simulink model "Interface_Model"  (R2017b)
settings: Solver=FixedStepDiscrete  StartTime=0.0  StopTime=inf  RelTol=1e-3  EnableMultiTasking=on
InitFcn:
  | modelSettings
undefined symbols (not defined in the file or in its folder): ip
libraries: gm_combinedTxRx_ExternalMode_lib x3
settings Model: SimulationMode=external  Creator=tcollins  LastModifiedBy=tcollins
settings SolverCC: PositivePriorityOrder=on
settings OptimizationCC: BlockReduction=off  ConditionallyExecuteInputs=off  PassReuseOutputArgsAs=Individual arguments  MaxStackSize=64
settings DebuggingCC: AlgebraicLoopMsg=error  SingleTaskRateTransMsg=error  ParameterTunabilityLossMsg=error
settings HardwareCC: ProdBitPerPointer=32  ProdBitPerSizeT=32  ProdBitPerPtrDiffT=32  ProdLargestAtomicInteger=Long  ProdLargestAtomicFloat=Double  ProdWordSize=32  ProdLongLongMode=on  ProdHWDeviceType=ARM Compatible->ARM Cortex  TargetLargestAtomicInteger=Long  TargetLargestAtomicFloat=Double  TargetIntDivRoundTo=Zero  TargetEndianess=LittleEndian  TargetHWDeviceType=ARM Compatible->ARM Cortex
settings SFSimCC: MATLABDynamicMemAlloc=off
settings RTWCC: SystemTargetFile=ert.tlc  HardwareBoard=Xilinx Zynq-7000 Based IIO Radio  TemplateMakefile=ert_default_tmf  Toolchain=Xilinx Software Development Kit (SDK)  IncludeHyperlinkInReport=on
settings CodeAppCC: ForceParamTrailComments=on  IgnoreCustomStorageClasses=off  OperatorAnnotations=on  SimulinkDataObjDesc=on  SFDataObjDesc=on  InsertBlockDesc=on

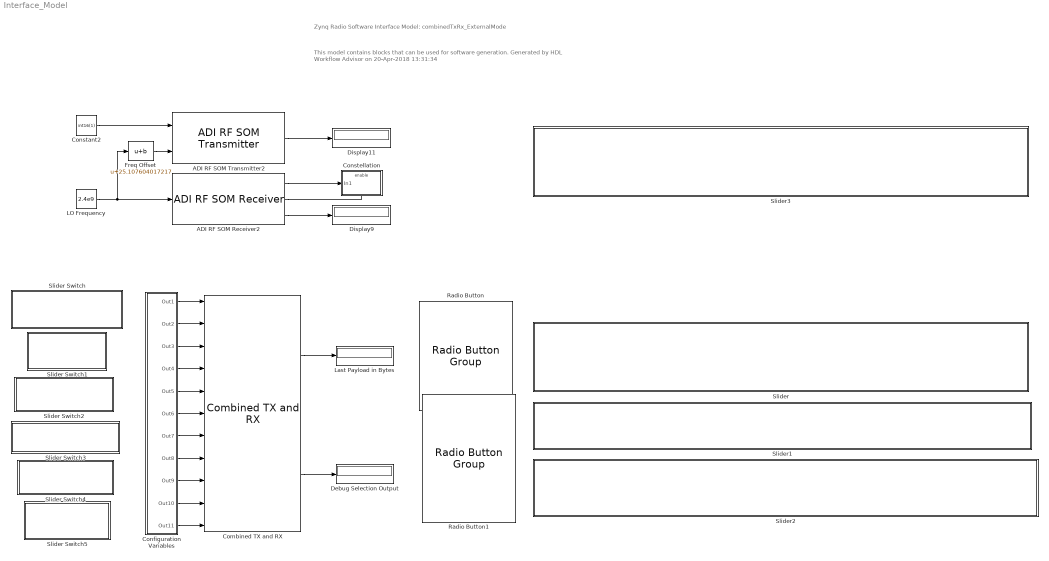
== system Interface_Model ==
  note: Zynq Radio Software Interface Model: combinedTxRx_ExternalMode
  note: This model contains blocks that can be used for software generation.
      |
      | Generated by HDL Workflow Advisor on 20-Apr-2018 13:31:34
  ADI RF SOM Receiver2 : gm_combinedTxRx_ExternalMode_lib/ADI RF SOM Receiver  IPAddress=192.168.3.2  uri=ip:10.0.0.200  CenterFrequencySource=Input Port  CenterFrequency=2.4e9  GainSource=AGC Slow Attack  Gain=10  ChannelMapping=1  BasebandSampleRate=1e6  OutputDataType=int16  SamplesPerFrame=20000  OverflowOutputPort=on  ShowAdvancedProperties=off  Timeout=30  EnableQuadratureTracking=on  EnableRFDCTracking=on  EnableBasebandDCTracking=on  UseCustomFilter=off  filtPathRates=[ 737280000, 11520000, 3840000, 1920000, 960000, 240000 ]  filtCoefficients=round( fir1( 127, 0.75 )*2^15*10^1.2 )  filtCoefficientSize=128  filtDecimInterpFactor=4  filtGain=-12  filtRFBandwidth=18e6  filterConfigStruct=struct()  ENSMPinControlMode=None  BISTLoopbackMode=Disabled
  ADI RF SOM Transmitter2 : gm_combinedTxRx_ExternalMode_lib/ADI RF SOM Transmitter  IPAddress=192.168.3.2  uri=ip:10.0.0.200  CenterFrequencySource=Input Port  CenterFrequency=2.4e9  GainSource=Dialog  Gain=-10  ChannelMapping=1  BasebandSampleRate=1e6  UnderflowOutputPort=on  ShowAdvancedProperties=off  Timeout=30  DataSourceSelect=Input Port  DDSTone1Freq=5e3  DDSTone2Freq=10e3  DDSTone1Scale=0.5  DDSTone2Scale=0.25  UseCustomFilter=off  filtPathRates=[ 737280000, 11520000, 3840000, 1920000, 960000, 240000 ]  filtCoefficients=round( fir1( 127, 0.75 )*2^15*10^1.2 )  filtCoefficientSize=128  filtDecimInterpFactor=4  filtGain=-12  filtRFBandwidth=18e6  filterConfigStruct=struct()  ENSMPinControlMode=None  BISTLoopbackMode=Disabled
  Combined TX and RX : gm_combinedTxRx_ExternalMode_lib/Combined TX and RX
  Configuration Variables : Subsystem
  Constant2 : Constant  Value=int16(1)  SampleTime=1/500
  Constellation : Subsystem
  Debug Selection Output : Display
  Display11 : Display
  Display9 : Display
  Freq Offset : Bias  Bias=25.107604017217
  LO Frequency : Constant  Value=2.4e9  SampleTime=1/500
  Last Payload in Bytes : Display
  Radio Button : RadioButtonGroup  WebBlockId=317  ModelName=Interface_Model  LabelPosition=Top  ShowInitialText=on  SelectedLabel=After Frequency Recovery  ButtonGroupName=Constellation Data Source
      settings: Values={{'After SRRC', 'After Timing Recovery', 'After Frequency Recovery', 'After EQ'}, [1 2 3 4]}
  Radio Button1 : RadioButtonGroup  WebBlockId=335  ModelName=Interface_Model  LabelPosition=Top  ShowInitialText=on  SelectedLabel=CRC Errors  ButtonGroupName=Constellation Data Source
      settings: Values={{'Timing Lock', 'Peaks Found', 'Freq Lock', 'Header Failures', 'CRC Errors', 'Packet Count', 'Last Payload Length'}, [0 1 2 3 4 5 6]}
  Slider : Subsystem  DialogController=hmiCreateDDGDialog  IsWebBlock=on  mask(MWDashboardBlock){webBlockId=d4feb81d-cb24-4eef-b536-d200a1891d41, webBlockType=slider, ShowInLibBrowser=on, ShowInitialText=on, HMISrcModelName=Interface_Model}
      mask prompts: webBlockId "WebBlock Id"; webBlockType "WebBlock Type"; HMISrcModelName "Source Model"
      mask help: SimulinkHMI:dialogs:SliderDialogDesc
      mask Help: helpview([docroot '/mapfiles/simulink.map'], 'hmi_slider')
      mask Display:
      | if strcmp(get_param(bdroot(gcb),'BlockDiagramType'), 'library')
      |     image([(matlabroot) '/toolbox/simulink/hmi/icons/Slider.png']);
      | end
  Slider Switch : Subsystem  DialogController=hmiCreateDDGDialog  IsWebBlock=on  mask(MWDashboardBlock){webBlockId=26219f1f-1109-40ca-a4af-2a8bc964a3a4, webBlockType=sliderswitch, ShowInLibBrowser=on, ShowInitialText=on, HMISrcModelName=Interface_Model}
      mask prompts: webBlockId "WebBlock Id"; webBlockType "WebBlock Type"; HMISrcModelName "Source Model"
      mask help: SimulinkHMI:dialogs:SwitchDialogDesc
      mask Help: helpview([docroot '/mapfiles/simulink.map'], 'hmi_slider_switch')
      mask Display:
      | if strcmp(get_param(bdroot(gcb),'BlockDiagramType'), 'library')
      |     image([(matlabroot) '/toolbox/simulink/hmi/icons/SliderSwitch.png']);
      | end
  Slider Switch1 : Subsystem  DialogController=hmiCreateDDGDialog  IsWebBlock=on  mask(MWDashboardBlock){webBlockId=1eddc475-4e28-4e7e-8fa4-3c106ebddf36, webBlockType=sliderswitch, ShowInLibBrowser=on, ShowInitialText=on, HMISrcModelName=Interface_Model}
      mask prompts: webBlockId "WebBlock Id"; webBlockType "WebBlock Type"; HMISrcModelName "Source Model"
      mask help: SimulinkHMI:dialogs:SwitchDialogDesc
      mask Help: helpview([docroot '/mapfiles/simulink.map'], 'hmi_slider_switch')
      mask Display:
      | if strcmp(get_param(bdroot(gcb),'BlockDiagramType'), 'library')
      |     image([(matlabroot) '/toolbox/simulink/hmi/icons/SliderSwitch.png']);
      | end
  Slider Switch2 : Subsystem  DialogController=hmiCreateDDGDialog  IsWebBlock=on  mask(MWDashboardBlock){webBlockId=eeafa1fd-631f-4ad5-a162-b269cb845515, webBlockType=sliderswitch, ShowInLibBrowser=on, ShowInitialText=on, HMISrcModelName=Interface_Model}
      mask prompts: webBlockId "WebBlock Id"; webBlockType "WebBlock Type"; HMISrcModelName "Source Model"
      mask help: SimulinkHMI:dialogs:SwitchDialogDesc
      mask Help: helpview([docroot '/mapfiles/simulink.map'], 'hmi_slider_switch')
      mask Display:
      | if strcmp(get_param(bdroot(gcb),'BlockDiagramType'), 'library')
      |     image([(matlabroot) '/toolbox/simulink/hmi/icons/SliderSwitch.png']);
      | end
  Slider Switch3 : Subsystem  DialogController=hmiCreateDDGDialog  IsWebBlock=on  mask(MWDashboardBlock){webBlockId=d26f103e-6633-4623-a5ec-df427e9233ad, webBlockType=sliderswitch, ShowInLibBrowser=on, ShowInitialText=on, HMISrcModelName=Interface_Model}
      mask prompts: webBlockId "WebBlock Id"; webBlockType "WebBlock Type"; HMISrcModelName "Source Model"
      mask help: SimulinkHMI:dialogs:SwitchDialogDesc
      mask Help: helpview([docroot '/mapfiles/simulink.map'], 'hmi_slider_switch')
      mask Display:
      | if strcmp(get_param(bdroot(gcb),'BlockDiagramType'), 'library')
      |     image([(matlabroot) '/toolbox/simulink/hmi/icons/SliderSwitch.png']);
      | end
  Slider Switch4 : Subsystem  DialogController=hmiCreateDDGDialog  IsWebBlock=on  mask(MWDashboardBlock){webBlockId=ba810177-532f-4366-b8e7-2a0e810ca864, webBlockType=sliderswitch, ShowInLibBrowser=on, ShowInitialText=on, HMISrcModelName=Interface_Model}
      mask prompts: webBlockId "WebBlock Id"; webBlockType "WebBlock Type"; HMISrcModelName "Source Model"
      mask help: SimulinkHMI:dialogs:SwitchDialogDesc
      mask Help: helpview([docroot '/mapfiles/simulink.map'], 'hmi_slider_switch')
      mask Display:
      | if strcmp(get_param(bdroot(gcb),'BlockDiagramType'), 'library')
      |     image([(matlabroot) '/toolbox/simulink/hmi/icons/SliderSwitch.png']);
      | end
  Slider Switch5 : Subsystem  DialogController=hmiCreateDDGDialog  IsWebBlock=on  mask(MWDashboardBlock){webBlockId=216110c8-cc91-453d-9952-97baaa76ee3d, webBlockType=sliderswitch, ShowInLibBrowser=on, ShowInitialText=on, HMISrcModelName=Interface_Model}
      mask prompts: webBlockId "WebBlock Id"; webBlockType "WebBlock Type"; HMISrcModelName "Source Model"
      mask help: SimulinkHMI:dialogs:SwitchDialogDesc
      mask Help: helpview([docroot '/mapfiles/simulink.map'], 'hmi_slider_switch')
      mask Display:
      | if strcmp(get_param(bdroot(gcb),'BlockDiagramType'), 'library')
      |     image([(matlabroot) '/toolbox/simulink/hmi/icons/SliderSwitch.png']);
      | end
  Slider1 : Subsystem  DialogController=hmiCreateDDGDialog  IsWebBlock=on  mask(MWDashboardBlock){webBlockId=ada10824-bcdc-457e-86db-13bcc653ecfd, webBlockType=slider, ShowInLibBrowser=on, ShowInitialText=on, HMISrcModelName=Interface_Model}
      mask prompts: webBlockId "WebBlock Id"; webBlockType "WebBlock Type"; HMISrcModelName "Source Model"
      mask help: SimulinkHMI:dialogs:SliderDialogDesc
      mask Help: helpview([docroot '/mapfiles/simulink.map'], 'hmi_slider')
      mask Display:
      | if strcmp(get_param(bdroot(gcb),'BlockDiagramType'), 'library')
      |     image([(matlabroot) '/toolbox/simulink/hmi/icons/Slider.png']);
      | end
  Slider2 : Subsystem  DialogController=hmiCreateDDGDialog  IsWebBlock=on  mask(MWDashboardBlock){webBlockId=948c7412-cd60-4ac0-9221-40aef6caa45a, webBlockType=slider, ShowInLibBrowser=on, ShowInitialText=on, HMISrcModelName=Interface_Model}
      mask prompts: webBlockId "WebBlock Id"; webBlockType "WebBlock Type"; HMISrcModelName "Source Model"
      mask help: SimulinkHMI:dialogs:SliderDialogDesc
      mask Help: helpview([docroot '/mapfiles/simulink.map'], 'hmi_slider')
      mask Display:
      | if strcmp(get_param(bdroot(gcb),'BlockDiagramType'), 'library')
      |     image([(matlabroot) '/toolbox/simulink/hmi/icons/Slider.png']);
      | end
  Slider3 : Subsystem  DialogController=hmiCreateDDGDialog  IsWebBlock=on  mask(MWDashboardBlock){webBlockId=89982bbb-9146-47d5-8233-539a33715bfc, webBlockType=slider, ShowInLibBrowser=on, ShowInitialText=on, HMISrcModelName=Interface_Model}
      mask prompts: webBlockId "WebBlock Id"; webBlockType "WebBlock Type"; HMISrcModelName "Source Model"
      mask help: SimulinkHMI:dialogs:SliderDialogDesc
      mask Help: helpview([docroot '/mapfiles/simulink.map'], 'hmi_slider')
      mask Display:
      | if strcmp(get_param(bdroot(gcb),'BlockDiagramType'), 'library')
      |     image([(matlabroot) '/toolbox/simulink/hmi/icons/Slider.png']);
      | end
  wires:
  Configuration Variables/2(Out2) -> Combined TX and RX/2
  Combined TX and RX/2 -> Debug Selection Output/1
  Configuration Variables/8(Out8) -> Combined TX and RX/8
  Configuration Variables/7(Out7) -> Combined TX and RX/7
  Configuration Variables/1(Out1) -> Combined TX and RX/1
  Configuration Variables/5(Out5) -> Combined TX and RX/5
  Configuration Variables/10(Out10) -> Combined TX and RX/10
  Configuration Variables/3(Out3) -> Combined TX and RX/3
  Configuration Variables/9(Out9) -> Combined TX and RX/9
  Configuration Variables/6(Out6) -> Combined TX and RX/6
  Combined TX and RX/1 -> Last Payload in Bytes/1
  Configuration Variables/4(Out4) -> Combined TX and RX/4
  Configuration Variables/11(Out11) -> Combined TX and RX/11
  ADI RF SOM Transmitter2/1 -> Display11/1
  ADI RF SOM Receiver2/3 -> Display9/1
  ADI RF SOM Receiver2/2 -> Constellation/Enable
  Constant2/1 -> ADI RF SOM Transmitter2/1
  ADI RF SOM Receiver2/1 -> Constellation/1(In1)
  LO Frequency/1 -> Freq Offset/1, ADI RF SOM Receiver2/1
  Freq Offset/1 -> ADI RF SOM Transmitter2/2

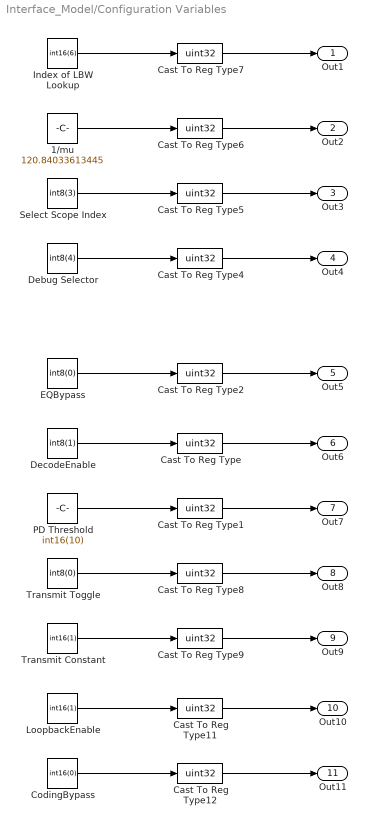
== system Interface_Model/Configuration Variables ==
  1/mu : Constant  Value=120.84033613445  OutDataTypeStr=int16  SampleTime=1/500
  Cast To Reg Type{,1..2,4..9,11..12} (11 alike) : DataTypeConversion  OutDataTypeStr=uint32
  CodingBypass : Constant  Value=int16(0)  SampleTime=1/500
  Debug Selector : Constant  Value=int8(4)  SampleTime=1/500
  DecodeEnable : Constant  Value=int8(1)  SampleTime=1/500
  EQBypass : Constant  Value=int8(0)  SampleTime=1/500
  Index of LBW Lookup : Constant  Value=int16(6)  SampleTime=1/500
  LoopbackEnable : Constant  Value=int16(1)  SampleTime=1/500
  PD Threshold : Constant  Value=int16(10)  SampleTime=1/500
  Select Scope Index : Constant  Value=int8(3)  SampleTime=1/500
  Transmit Constant : Constant  Value=int16(1)  SampleTime=1/500
  Transmit Toggle : Constant  Value=int8(0)  SampleTime=1/500
  Out1 : Outport
  Out2 : Outport  Port=2
  Out3 : Outport  Port=3
  Out4 : Outport  Port=4
  Out5 : Outport  Port=5
  Out6 : Outport  Port=6
  Out7 : Outport  Port=7
  Out8 : Outport  Port=8
  Out9 : Outport  Port=9
  Out10 : Outport  Port=10
  Out11 : Outport  Port=11
  wires:
  1/mu/1 -> Cast To Reg Type6/1
  Index of LBW Lookup/1 -> Cast To Reg Type7/1
  Select Scope Index/1 -> Cast To Reg Type5/1
  Debug Selector/1 -> Cast To Reg Type4/1
  EQBypass/1 -> Cast To Reg Type2/1
  DecodeEnable/1 -> Cast To Reg Type/1
  PD Threshold/1 -> Cast To Reg Type1/1
  Cast To Reg Type1/1 -> Out7/1
  Cast To Reg Type/1 -> Out6/1
  Cast To Reg Type2/1 -> Out5/1
  Cast To Reg Type4/1 -> Out4/1
  Cast To Reg Type5/1 -> Out3/1
  Cast To Reg Type6/1 -> Out2/1
  Cast To Reg Type7/1 -> Out1/1
  Transmit Toggle/1 -> Cast To Reg Type8/1
  Transmit Constant/1 -> Cast To Reg Type9/1
  Cast To Reg Type9/1 -> Out9/1
  Cast To Reg Type8/1 -> Out8/1
  LoopbackEnable/1 -> Cast To Reg Type11/1
  Cast To Reg Type11/1 -> Out10/1
  CodingBypass/1 -> Cast To Reg Type12/1
  Cast To Reg Type12/1 -> Out11/1

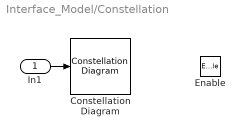
== system Interface_Model/Constellation ==
  In1 : Inport
  Enable : EnablePort
  Constellation Diagram : ConstellationDiagram
  wires:
  In1/1 -> Constellation Diagram/1

== system Interface_Model/Slider ==

== system Interface_Model/Slider Switch ==

== system Interface_Model/Slider Switch1 ==

== system Interface_Model/Slider Switch2 ==

== system Interface_Model/Slider Switch3 ==

== system Interface_Model/Slider Switch4 ==

== system Interface_Model/Slider Switch5 ==

== system Interface_Model/Slider1 ==

== system Interface_Model/Slider2 ==

== system Interface_Model/Slider3 ==
